simulink model "kette3mOhneCallBack"  (R2018b)
settings: Solver=FixedStepAuto  StartTime=0.0  StopTime=20.0  FixedStep=0.1  MaxStep=0.1  MinStep=0.1  RelTol=1e-3  EnableMultiTasking=on
values from neighbouring files (symbols this model uses):
  c1 = c    (= 1)    [setParamKette3m.m]
  c2 = c    (= 1)    [setParamKette3m.m]
  c3 = c    (= 1)    [setParamKette3m.m]
  c4 = c    (= 1)    [setParamKette3m.m]
  m1 = m    (= 2)    [setParamKette3m.m]
  m2 = m    (= 2)    [setParamKette3m.m]
  m3 = m    (= 2)    [setParamKette3m.m]
  v10 = 0    [setParamKette3m.m]
  v20 = 0    [setParamKette3m.m]
  v30 = 0    [setParamKette3m.m]
  x10 = -1    [setParamKette3m.m]
  x20 = 0    [setParamKette3m.m]
  x30 = 1    [setParamKette3m.m]
undefined symbols (not defined in the file or in its folder): v1, v2, v3, x1, x2, x3
settings Model: Creator=Reichl  LastModifiedBy=Reichl
settings DataIOCC: SaveFormat=Array  SignalLoggingSaveFormat=ModelDataLogs
settings OptimizationCC: ExpressionDepthLimit=2147483647  LifeSpan=inf
settings DebuggingCC: UnderspecifiedInitializationDetection=Classic  MergeDetectMultiDrivingBlocksExec=none  SolverPrmCheckMsg=warning  FcnCallInpInsideContextMsg=warning  AllowSymbolicDim=off  StateNameClashWarn=warning  SFUnexpectedBacktrackingDiag=warning  SFNoUnconditionalDefaultTransitionDiag=warning  SFExecutionAtInitializationDiag=none
settings HardwareCC: ProdBitPerPointer=32  ProdBitPerSizeT=32  ProdBitPerPtrDiffT=32  ProdLargestAtomicFloat=None  ProdIntDivRoundTo=Undefined  ProdEndianess=Unspecified  ProdWordSize=32  ProdHWDeviceType=32-bit Generic
settings ModelReferenceCC: PropagateSignalLabelsOutOfModel=off
settings SFSimCC: SimUseLocalCustomCode=off
settings RTWCC: RTWUseLocalCustomCode=off
settings CodeAppCC: StateflowObjectComments=on
settings GRTTargetCC: TargetLangStandard=C89/C90 (ANSI)  GeneratePreprocessorConditionals=Disable all  CombineOutputUpdateFcns=off  GRTInterface=on
settings ConfigComp: CovMetricSettings=dw  CovHtmlReporting=on  CovSaveCumulativeToWorkspaceVar=on  CovSaveSingleToWorkspaceVar=on  CovExternalEMLEnable=off  CovSFcnEnable=off

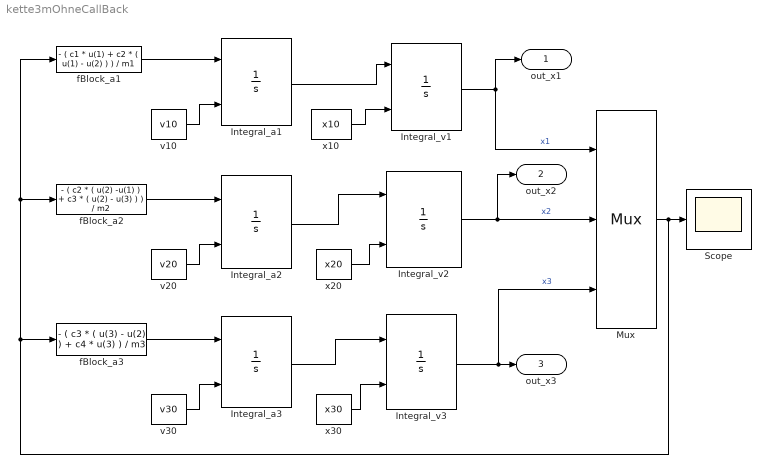
== system kette3mOhneCallBack ==
  Integral_a1 : Integrator  InitialConditionSource=external  InitialCondition=v1
  Integral_a2 : Integrator  InitialConditionSource=external  InitialCondition=v2
  Integral_a3 : Integrator  InitialConditionSource=external  InitialCondition=v3
  Integral_v1 : Integrator  InitialConditionSource=external  InitialCondition=x1
  Integral_v2 : Integrator  InitialConditionSource=external  InitialCondition=x2
  Integral_v3 : Integrator  InitialConditionSource=external  InitialCondition=x3
  Mux : Mux  Inputs=3
      settings: DisplayOption=signals
  Scope : Scope
  fBlock_a1 : Fcn  Expr="- (   c1 * u(1)  +  c2 * ( u(1) - u(2) )  ) / m1"
  fBlock_a2 : Fcn  Expr="- (   c2 * ( u(2)  -u(1) )  +  c3 * ( u(2) - u(3) )  ) / m2"
  fBlock_a3 : Fcn  Expr="- (  c3 * ( u(3) - u(2) )  +  c4 * u(3)  ) / m3"
  v10 : Constant  Value=v10
  v20 : Constant  Value=v20
  v30 : Constant  Value=v30
  x10 : Constant  Value=x10
  x20 : Constant  Value=x20
  x30 : Constant  Value=x30
  out_x1 : Outport
  out_x2 : Outport  Port=2
  out_x3 : Outport  Port=3
  wires:
  Integral_a1/1 -> Integral_v1/1
  Integral_a2/1 -> Integral_v2/1
  Integral_a3/1 -> Integral_v3/1
  Mux/1 -> Scope/1, fBlock_a1/1, fBlock_a2/1, fBlock_a3/1
  Integral_v2/1 -> out_x2/1, Mux/2  "x2"
  Integral_v1/1 -> out_x1/1, Mux/1  "x1"
  Integral_v3/1 -> out_x3/1, Mux/3  "x3"
  fBlock_a1/1 -> Integral_a1/1
  fBlock_a2/1 -> Integral_a2/1
  fBlock_a3/1 -> Integral_a3/1
  v10/1 -> Integral_a1/2
  v20/1 -> Integral_a2/2
  v30/1 -> Integral_a3/2
  x10/1 -> Integral_v1/2
  x30/1 -> Integral_v3/2
  x20/1 -> Integral_v2/2
